simulink model "SMC_for_nonlinear_system"  (Simulink 9.3)
settings: Solver=FixedStepAuto  StartTime=0.0  StopTime=20  FixedStep=0.01  RelTol=1e-3
settings Model: Creator=User2  LastModifiedBy=User2
settings DataIOCC: SaveFormat=Dataset  SignalLoggingSaveFormat=Dataset  ReturnWorkspaceOutputs=on
settings OptimizationCC: LifeSpan=auto
settings DebuggingCC: UnderspecifiedInitializationDetection=Simplified  MergeDetectMultiDrivingBlocksExec=error  FcnCallInpInsideContextMsg=error  SFUnexpectedBacktrackingDiag=error  SFNoUnconditionalDefaultTransitionDiag=error  SFExecutionAtInitializationDiag=warning  ArithmeticOperatorsInVariantConditions=error
settings HardwareCC: ProdBitPerPointer=64  ProdBitPerSizeT=64  ProdBitPerPtrDiffT=64  ProdLargestAtomicFloat=Float  ProdIntDivRoundTo=Zero  ProdEndianess=LittleEndian  ProdWordSize=64  ProdHWDeviceType=Intel->x86-64 (Windows64)
settings ModelReferenceCC: PropagateSignalLabelsOutOfModel=on
settings SFSimCC: SimUseLocalCustomCode=on
settings RTWCC: RTWUseLocalCustomCode=on
settings CodeAppCC: StateflowObjectComments=off
settings GRTTargetCC: TargetLangStandard=C99 (ISO)  CombineOutputUpdateFcns=on  GRTInterface=off
settings ConfigComp: CovMetricSettings=dwe  CovHtmlReporting=off  CovSaveCumulativeToWorkspaceVar=off  CovSaveSingleToWorkspaceVar=off  CovExternalEMLEnable=on

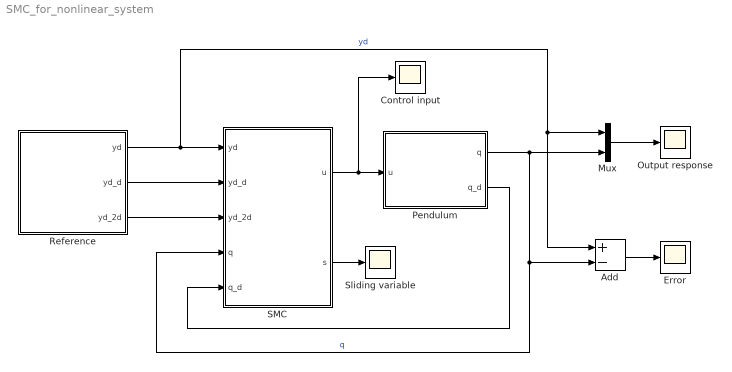
== system SMC_for_nonlinear_system ==
  Add : Sum  Inputs=+-
  Control input : Scope
  Error : Scope
  Mux : Mux  Inputs=2
  Output response : Scope
  Pendulum : Subsystem
  Reference : Subsystem
  SMC : MATLAB Function  TreatAsAtomicUnit=on
  Sliding variable : Scope
  wires:
  SMC/1(u) -> Pendulum/1(u), Control input/1
  Reference/1(yd) -> SMC/1(yd), Add/1, Mux/1  "yd"
  Reference/2(yd_d) -> SMC/2(yd_d)
  Reference/3(yd_2d) -> SMC/3(yd_2d)
  Mux/1 -> Output response/1
  Add/1 -> Error/1
  SMC/2(s) -> Sliding variable/1
  Pendulum/1(q) -> SMC/4(q), Add/2, Mux/2  "q"
  Pendulum/2(q_d) -> SMC/5(q_d)

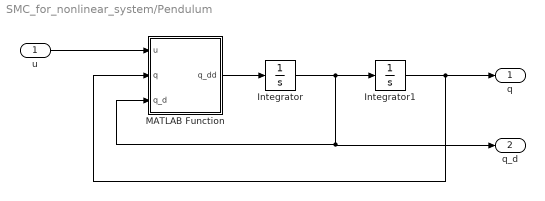
== system SMC_for_nonlinear_system/Pendulum ==
  u : Inport
  Integrator : Integrator
  Integrator1 : Integrator
  MATLAB Function : MATLAB Function  TreatAsAtomicUnit=on
  q : Outport
  q_d : Outport  Port=2
  wires:
  u/1 -> MATLAB Function/1(u)
  MATLAB Function/1(q_dd) -> Integrator/1
  Integrator/1 -> Integrator1/1, q_d/1, MATLAB Function/3(q_d)
  Integrator1/1 -> q/1, MATLAB Function/2(q)

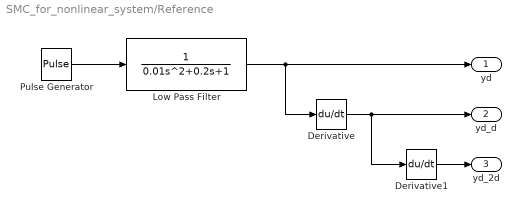
== system SMC_for_nonlinear_system/Reference ==
  Derivative : Derivative
  Derivative1 : Derivative
  Low Pass Filter : TransferFcn  Denominator=[0.01 0.2 1]
  Pulse Generator : DiscretePulseGenerator  PulseType=Time based  Amplitude=pi/3  Period=20  PulseWidth=50
  yd : Outport
  yd_d : Outport  Port=2
  yd_2d : Outport  Port=3
  wires:
  Pulse Generator/1 -> Low Pass Filter/1
  Low Pass Filter/1 -> Derivative/1, yd/1
  Derivative/1 -> Derivative1/1, yd_d/1
  Derivative1/1 -> yd_2d/1

== matlab function Pendulum/MATLAB Function ==
  data: u input double; q input double; q_dd output double; q_d input double
function q_dd = Pendulum(u, q, q_d)
%% Declaration
m=0.1; 
l=1; 
B=0.01;
g=9.81;
d=0.2*sign(q_d);

gg=1/(m*l^2);
d1=-gg*d;
f=-g/l*sin(q)-B/(m*l^2)*q_d;

%% Simulation
q_dd=f+gg*u+d1;
%%q_dd=1/(m*l^2)*(u-B*q_d-m*g*l*sin(q)-0.2*sign(q_d));

== matlab function SMC ==
  data: yd input double; yd_d input double; yd_2d input double; u output double; q input double; q_d input double; s output double
function [u,s]= SMC(yd, yd_d, yd_2d, q, q_d)
%% Declaration
m=0.1;
l=1;
B=0.01;
g=9.81;
lamda=10;
k=20;
eta=2;

f=-g/l*sin(q)-B/(m*l^2)*q_d;
gg=1/(m*l^2);

e=q-yd;
e_d=q_d-yd_d;
s=e_d+lamda*e;

%% Control output
u=(1/gg)*(yd_2d-lamda*e_d-f-k*s-eta*sign(s));
